simulink model "Planta_completa_expandida_controle_velocidade"  (R2023b)
settings: Solver=VariableStepAuto  StartTime=0.0  StopTime=7  RelTol=1e-3
model workspace (MAT data in the model file):
  B = 0.0928996133407
  Cmn = 479.991198073
  I = 3000
  Ian = 260.13143483
  J = 0.56
  Kf = 1.91586963478
  La = 0.0014
  N = 3000
  Pele = 104052.573932
  Pmec = 95000
  Ra = 0.08
  T = 0.00175
  Te = 0.0175
  Tm = 6.02801217209
  Vn = 400
  Wn = 197.920296
libraries: simulink x2
settings Model: Creator=lpds  LastModifiedBy=lpds

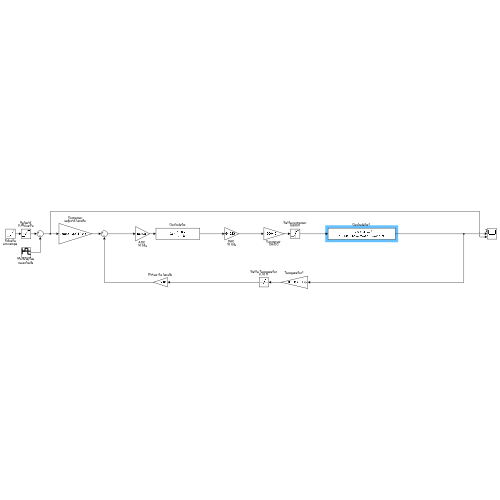
[thumbnail: Simulink's stored preview of the top-level diagram]
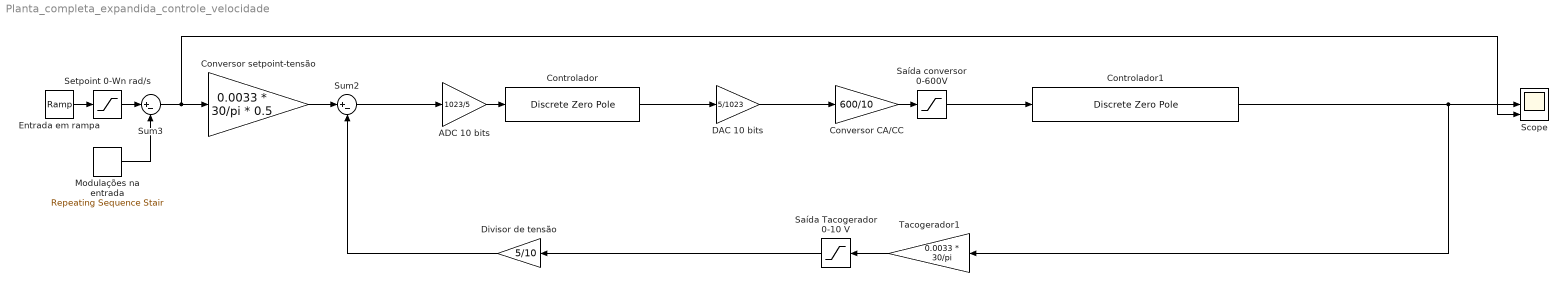
== system Planta_completa_expandida_controle_velocidade ==
  "ADC 10 bits " : Gain  Gain=1023/5
  Controlador : DiscreteZeroPole  Zeros=[0.9]  Poles=[1]  Gain=0.1  SampleTime=T
  Controlador1 : DiscreteZeroPole  Zeros=[0.005854 0 0]  Poles=[1 1.9224928 0.9337476]  Gain=1  SampleTime=T
  Conversor setpoint-tensão : Gain  Gain=0.0033 * 30/pi * 0.5
  Conversor CA/CC : Gain  Gain=600/10
  DAC 10 bits : Gain  Gain=5/1023
  Divisor de tensão : Gain  Gain=5/10
  Entrada em rampa : simulink/Sources/Ramp  slope=Wn*2  start=0  InitialOutput=0
  Modulações na entrada : simulink/Sources/Repeating Sequence Stair  OutValues=[0 50 -50].'  tsamp=1143 * 0.00175  OutMin=[]  OutMax=[]  OutDataTypeStr=double  OutputDataTypeScalingMode=double  OutDataType=fixdt(0,8)  ConRadixGroup=Best Precision: Vector-wise  OutScaling=2^-12
  Saída Tacogerador 0-10 V : Saturate  UpperLimit=10  LowerLimit=0
  Saída conversor 0-600V : Saturate  UpperLimit=600  LowerLimit=0
  Scope : Scope  NumInputPorts=3
  Setpoint 0-Wn rad/s : Saturate  UpperLimit=Wn
  Sum2 : Sum  Inputs=|+-
  Sum3 : Sum  Inputs=|+-
  Tacogerador1 : Gain  Gain=0.0033 * 30/pi
  wires:
  Saída Tacogerador 0-10 V/1 -> Divisor de tensão/1
  Saída conversor 0-600V/1 -> Controlador1/1
  Conversor CA/CC/1 -> Saída conversor 0-600V/1
  DAC 10 bits/1 -> Conversor CA/CC/1
  Controlador/1 -> DAC 10 bits/1
  Sum3/1 -> Scope/3, Conversor setpoint-tensão/1
  Conversor setpoint-tensão/1 -> Sum2/1
  "ADC 10 bits "/1 -> Controlador/1
  Sum2/1 -> "ADC 10 bits "/1
  Divisor de tensão/1 -> Sum2/2
  Setpoint 0-Wn rad/s/1 -> Sum3/1
  Entrada em rampa/1 -> Setpoint 0-Wn rad/s/1
  Tacogerador1/1 -> Saída Tacogerador 0-10 V/1
  Controlador1/1 -> Tacogerador1/1, Scope/2
  Modulações na entrada/1 -> Sum3/2
